simulink model "simulateDBPSK"  (R2017a)
settings: Solver=VariableStepAuto  StartTime=0.0  StopTime=1  RelTol=1e-3
libraries: commdigbbndpm3 x2, commchan3 x1, commrandsrc3 x1, commsink2 x1, commrflib2 x1
settings Model: Creator=prust  LastModifiedBy=prust

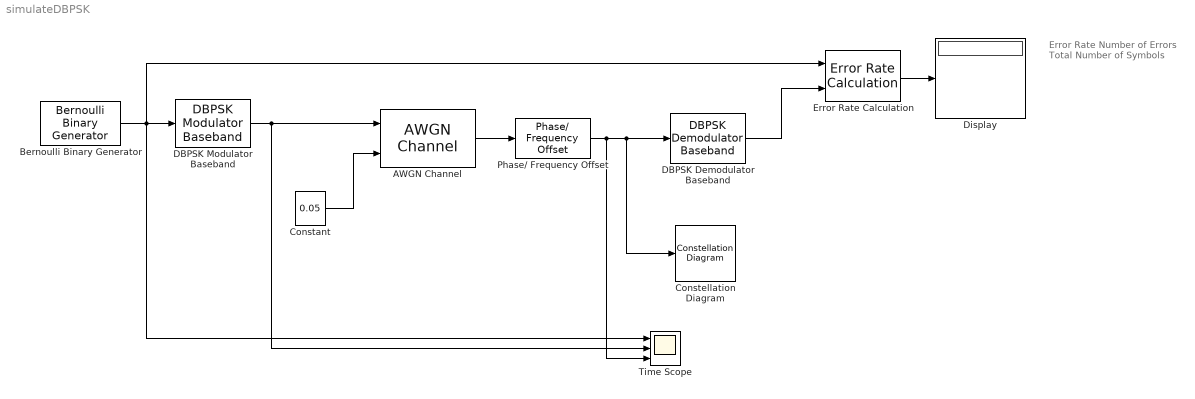
== system simulateDBPSK ==
  note: Error Rate
      |
      | Number of Errors
      |
      | Total Number of Symbols
  AWGN Channel : commchan3/AWGN Channel  InputProcessing=Columns as channels (frame based)  seed=67  noiseMode=Variance from port  EbNodB=50  EsNodB=10  SNRdB=10  bitsPerSym=1  Ps=1  Tsym=1/8000  variance=1
  Bernoulli Binary Generator : commrandsrc3/Bernoulli Binary Generator  ProbabilityOfZero=0.5  SeedSource=Auto  Seed=0  SampleTime=1/8000  SamplesPerFrame=1000  OutputDataType=double  SimulateUsing=Interpreted execution
  Constant : Constant  Value=0.05  VectorParams1D=off
  Constellation Diagram : ConstellationDiagram
  DBPSK Demodulator Baseband : commdigbbndpm3/DBPSK Demodulator Baseband  Ph=0  outDtype=Inherit via internal rule
      settings: SourceProductName=Communications System Toolbox  SourceProductBaseCode=CM
  DBPSK Modulator Baseband : commdigbbndpm3/DBPSK Modulator Baseband  Ph=0  outDtype=double
      settings: SourceProductName=Communications System Toolbox  SourceProductBaseCode=CM
  Display : Display
  Error Rate Calculation : commsink2/Error Rate Calculation  N=0  st_delay=0  cp_mode=Entire frame  subframe=[]  PMode=Port  WsName=ErrorVec  RsMode2=off  stop=off  numErr=100  maxBits=1e6
  Phase/ Frequency Offset : commrflib2/Phase// Frequency Offset  phaseOffset=30  freqPort=off  freqOffset=0
      settings: SourceProductName=Communications System Toolbox
  Time Scope : Scope  NumInputPorts=3
  wires:
  Bernoulli Binary Generator/1 -> DBPSK Modulator Baseband/1, Time Scope/1, Error Rate Calculation/1
  DBPSK Modulator Baseband/1 -> AWGN Channel/1, Time Scope/2
  AWGN Channel/1 -> Phase/ Frequency Offset/1
  DBPSK Demodulator Baseband/1 -> Error Rate Calculation/2
  Error Rate Calculation/1 -> Display/1
  Phase/ Frequency Offset/1 -> Time Scope/3, Constellation Diagram/1, DBPSK Demodulator Baseband/1
  Constant/1 -> AWGN Channel/2
